simulink model "PubIfDecisionTOS_MDL"  (R2020b)
settings: configuration reference "DspaceConfig" (kept outside this file)
PostLoadFcn:
  | if any(exist('dsrtsu_mdlpostloadfcn', 'file') ~= 0), dsrtsu_mdlpostloadfcn('Execute', bdroot); end
InitFcn:
  | , if any(exist('dsmpb_private', 'file') ~= 0), dsmpb_private('dsmpb_mdlclblib', 'Init', bdroot); end,
undefined symbols (not defined in the file or in its folder): C_TOS_ACCEgoRAxletoFbumplength_m, C_TOS_ACCTargetFront_Flag, C_TOS_AEBJAPedObjDxThre_Val, C_TOS_AEBJAPedObjDyThre_Val, C_TOS_AEBJATargetSize_Val, C_TOS_AEBJAVehObjDxThre_Val, C_TOS_AEBJAVehObjDyThre_Val, C_TOS_AEBJuncPedTargetSize_Val, C_TOS_AEBLatObjDxThre_Val, C_TOS_AEBLatPedDyThre_Val, C_TOS_AEBLatTargetSize_Val, C_TOS_AEBLongTargetInEgoFront_Flag, C_TOS_axAbsGround_Parameter, C_TOS_CameraConfirmedFlag, C_TOS_CNsubjWidth, C_TOS_CurrentLaneCoreMinWidth_Val, C_TOS_CutInProb_Val_Zero, C_TOS_CutOutProb_Val_Zero, C_TOS_D2R_Val, C_TOS_DefaultValueObjectToCenterLine_dy, C_TOS_EgoCarWidth_Val, C_TOS_EgoDxRefPoint_m, C_TOS_EgoRAxletoFbumplength_m, C_TOS_HalfWidthVehicle_Con, C_TOS_HWA_CurrentLaneFlag, C_TOS_HWA_LeftLaneFlag, C_TOS_HWA_MovingDir_Vaild, C_TOS_HWA_MovState_Vaild, C_TOS_HWA_RightLaneFlag, C_TOS_LaneLineCourseErrorFront, C_TOS_LaneLineCourseErrorRear, C_TOS_MotorbikeDefaultWidth_m, C_TOS_NumberOfEffectiveTargets, C_TOS_Obj_Age_Val, C_TOS_Objdx_Constraint_Val, C_TOS_ObjectDefaultWidth_m, C_TOS_ObjInCurrentLane_Val, C_TOS_ObjInCurrentLaneValid, C_TOS_ObjInLeftLaneValid, C_TOS_ObjInRightLaneValid, C_TOS_ObjNotInCurrentLane_Val, C_TOS_ObjNotREElementType, C_TOS_ObjPredictDis_dy_ConstantVal_Zeros, C_TOS_ObjToCenterLine_ConstantVal_Zeros, C_TOS_OFMObjIDInvilad_Val, C_TOS_PIL_LatDisCons_Val_zero, C_TOS_PIL_ObjectCutInFlag_b, C_TOS_PIL_ObjectCutOutFlag_b, C_TOS_PIL_ObjLaneProb_al_Val, C_TOS_PP_ObjFusType_FC_Confirm_b, C_TOS_PP_ObjFusType_FC_FR_Confirm_b, C_TOS_PP_ObjFusType_FR_Confirm_b, C_TOS_RE_80BoolDefault_Val, C_TOS_RE_80Single181Default_Val, C_TOS_RE_80Single255Default_Val, C_TOS_RE_80Uint8Default_Val, C_TOS_RE_D2R, C_TOS_RE_D_180_Val, C_TOS_RE_InvalidObjectID_Val, C_TOS_RE_InvalidTargetChainDir_Val ... (+142)
libraries: simulink x1650, TOS_LIB x361, canfdmsglib x14
(part 29 of 69)

== system PubIfDecisionTOS_MDL/TOS_20201112/TOS_2012080320/TOS/AEB/TOS_AEBJunct_20201208/AEBJunc_Object_Condition1/AEBJA_TargetCondition/TOS_AEBJunc_TargetsCondition ==
  Object_ID : Inport
  PP_ObjFusType_FC_FR_Confirm : Inport  Port=2
  PP_ObjFusType_FR_Confirm : Inport  Port=3
  ObjectType : Inport  Port=4
  Object_Dx : Inport  Port=5
  Object_Dy : Inport  Port=6
  PP_ObjMovingDirSignalProcessing : Inport  Port=7
  Object_HeadingAngle : Inport  Port=8
  Object_VX : Inport  Port=9
  Object_VY : Inport  Port=10
  VIE_EgoVelocity : Inport  Port=11
  psiDtOpt : Inport  Port=12
  axvRefMs2 : Inport  Port=13
  Object_MovingState : Inport  Port=14
  AEBJunc_Target_ObjectID_K1 : Inport  Port=15
  AEBJunc_Target_ObjectType_K1 : Inport  Port=16
  Action Port : ActionPort
  AEBJunc_PedTargetCondition : Subsystem
  AEBJunc_VehTargetCondition : Subsystem
  Bus Creator : BusCreator  Inputs=16
  Bus Selector : BusSelector  OutputSignals=Object_ID,PP_ObjFusType_FC_FR_Confirm,PP_ObjFusType_FR_Confirm,ObjectType,Object_Dx,Object_Dy,PP_ObjMovingDirSignalProcessing,Object_HeadingAngle,Object_VX,Object_VY,VIE_EgoVelocity,psiDtOpt,axvRefMs2,AEBJunc_Target_ObjectID_K1,AEBJunc_Target_ObjectType_K1
  Bus Selector1 : BusSelector  OutputSignals=Object_ID,PP_ObjFusType_FC_FR_Confirm,PP_ObjFusType_FR_Confirm,ObjectType,Object_Dx,Object_Dy,PP_ObjMovingDirSignalProcessing,Object_HeadingAngle,Object_VX,Object_VY,VIE_EgoVelocity,psiDtOpt,axvRefMs2,AEBJunc_Target_ObjectID_K1,AEBJunc_Target_ObjectType_K1,Object_MovingState
  TOS_AEBJunc_PedTargetsDx : Outport
  TOS_AEBJunc_VehTargetsDx : Outport  Port=2
  AEBJunc_PedTargetFusionType_observal : Outport  Port=3
  AEBJunc_PedTargetObjectType_observal : Outport  Port=4
  AEBJunc_PedTargetDXDY_observal : Outport  Port=5
  AEBJunc_PedTargetMovDir_observal : Outport  Port=6
  AEBJunc_VehTargetFusionType_observal : Outport  Port=7
  AEBJunc_VehTargetObjectType_observal : Outport  Port=8
  AEBJunc_VehTargetDXDY_observal : Outport  Port=9
  AEBJunc_VehTargetMovDir_observal : Outport  Port=10
  AEBJunc_VehTargetMovState_observal : Outport  Port=11
  wires:
  AEBJunc_VehTargetCondition/6(AEBJunc_VehTargetMovState_observal) -> AEBJunc_VehTargetMovState_observal/1
  Bus Selector1/16 -> AEBJunc_VehTargetCondition/16(Object_MovingState)  "<Object_MovingState>"
  Object_MovingState/1 -> Bus Creator/14  "Object_MovingState"
  AEBJunc_VehTargetCondition/1(TOS_AEBJunc_VehTargetsDx) -> TOS_AEBJunc_VehTargetsDx/1
  AEBJunc_VehTargetCondition/2(AEBJunc_VehTargetFusionType_observal) -> AEBJunc_VehTargetFusionType_observal/1
  AEBJunc_VehTargetCondition/3(AEBJunc_VehTargetObjectType_observal) -> AEBJunc_VehTargetObjectType_observal/1
  AEBJunc_VehTargetCondition/4(AEBJunc_VehTargetDXDY_observal) -> AEBJunc_VehTargetDXDY_observal/1
  AEBJunc_VehTargetCondition/5(AEBJunc_VehTargetMovDir_observal) -> AEBJunc_VehTargetMovDir_observal/1
  Bus Selector1/1 -> AEBJunc_VehTargetCondition/1(Object_ID)  "<Object_ID>"
  Bus Selector1/2 -> AEBJunc_VehTargetCondition/2(PP_ObjFusType_FC_FR_Confirm)  "<PP_ObjFusType_FC_FR_Confirm>"
  Bus Selector1/3 -> AEBJunc_VehTargetCondition/3(PP_ObjFusType_FR_Confirm)  "<PP_ObjFusType_FR_Confirm>"
  Bus Selector1/4 -> AEBJunc_VehTargetCondition/4(ObjectType)  "<ObjectType>"
  Bus Selector1/5 -> AEBJunc_VehTargetCondition/5(Object_Dx)  "<Object_Dx>"
  Bus Selector1/6 -> AEBJunc_VehTargetCondition/6(Object_Dy)  "<Object_Dy>"
  Bus Selector1/7 -> AEBJunc_VehTargetCondition/7(PP_ObjMovingDirSignalProcessing)  "<PP_ObjMovingDirSignalProcessing>"
  Bus Selector1/8 -> AEBJunc_VehTargetCondition/8(Object_HeadingAngle)  "<Object_HeadingAngle>"
  Bus Selector1/9 -> AEBJunc_VehTargetCondition/9(Object_VX)  "<Object_VX>"
  Bus Selector1/10 -> AEBJunc_VehTargetCondition/10(Object_VY)  "<Object_VY>"
  Bus Selector1/11 -> AEBJunc_VehTargetCondition/11(VIE_EgoVelocity)  "<VIE_EgoVelocity>"
  Bus Selector1/12 -> AEBJunc_VehTargetCondition/12(psiDtOpt)  "<psiDtOpt>"
  Bus Selector1/13 -> AEBJunc_VehTargetCondition/13(axvRefMs2)  "<axvRefMs2>"
  Bus Selector1/14 -> AEBJunc_VehTargetCondition/14(AEBJunc_VehTarget_ObjectID_K1)  "<AEBJunc_Target_ObjectID_K1>"
  Bus Selector1/15 -> AEBJunc_VehTargetCondition/15(AEBJunc_Target_ObjectType_K1)  "<AEBJunc_Target_ObjectType_K1>"
  Bus Selector/15 -> AEBJunc_PedTargetCondition/15(AEBJunc_Target_ObjectType_K1)  "<AEBJunc_Target_ObjectType_K1>"
  Bus Selector/14 -> AEBJunc_PedTargetCondition/14(AEBJunc_PedTarget_ObjectID_K1)  "<AEBJunc_Target_ObjectID_K1>"
  Bus Selector/13 -> AEBJunc_PedTargetCondition/13(axvRefMs2)  "<axvRefMs2>"
  Bus Selector/12 -> AEBJunc_PedTargetCondition/12(psiDtOpt)  "<psiDtOpt>"
  Bus Selector/11 -> AEBJunc_PedTargetCondition/11(VIE_EgoVelocity)  "<VIE_EgoVelocity>"
  Bus Selector/10 -> AEBJunc_PedTargetCondition/10(Object_VY)  "<Object_VY>"
  Bus Selector/9 -> AEBJunc_PedTargetCondition/9(Object_VX)  "<Object_VX>"
  Bus Selector/8 -> AEBJunc_PedTargetCondition/8(Object_HeadingAngle)  "<Object_HeadingAngle>"
  Bus Selector/7 -> AEBJunc_PedTargetCondition/7(PP_ObjMovingDirSignalProcessing)  "<PP_ObjMovingDirSignalProcessing>"
  Bus Selector/6 -> AEBJunc_PedTargetCondition/6(Object_Dy)  "<Object_Dy>"
  Bus Selector/5 -> AEBJunc_PedTargetCondition/5(Object_Dx)  "<Object_Dx>"
  Bus Selector/4 -> AEBJunc_PedTargetCondition/4(ObjectType)  "<ObjectType>"
  Bus Selector/3 -> AEBJunc_PedTargetCondition/3(PP_ObjFusType_FR_Confirm)  "<PP_ObjFusType_FR_Confirm>"
  Bus Selector/2 -> AEBJunc_PedTargetCondition/2(PP_ObjFusType_FC_FR_Confirm)  "<PP_ObjFusType_FC_FR_Confirm>"
  Bus Selector/1 -> AEBJunc_PedTargetCondition/1(Object_ID)  "<Object_ID>"
  Bus Creator/1 -> Bus Selector/1, Bus Selector1/1
  AEBJunc_Target_ObjectType_K1/1 -> Bus Creator/16  "AEBJunc_Target_ObjectType_K1"
  AEBJunc_Target_ObjectID_K1/1 -> Bus Creator/15  "AEBJunc_Target_ObjectID_K1"
  axvRefMs2/1 -> Bus Creator/13  "axvRefMs2"
  psiDtOpt/1 -> Bus Creator/12  "psiDtOpt"
  VIE_EgoVelocity/1 -> Bus Creator/11  "VIE_EgoVelocity"
  Object_VY/1 -> Bus Creator/10  "Object_VY"
  Object_VX/1 -> Bus Creator/9  "Object_VX"
  Object_HeadingAngle/1 -> Bus Creator/8  "Object_HeadingAngle"
  PP_ObjMovingDirSignalProcessing/1 -> Bus Creator/7  "PP_ObjMovingDirSignalProcessing"
  Object_Dy/1 -> Bus Creator/6  "Object_Dy"
  Object_Dx/1 -> Bus Creator/5  "Object_Dx"
  ObjectType/1 -> Bus Creator/4  "ObjectType"
  PP_ObjFusType_FR_Confirm/1 -> Bus Creator/3  "PP_ObjFusType_FR_Confirm"
  PP_ObjFusType_FC_FR_Confirm/1 -> Bus Creator/2  "PP_ObjFusType_FC_FR_Confirm"
  Object_ID/1 -> Bus Creator/1  "Object_ID"
  AEBJunc_PedTargetCondition/5(AEBJunc_PedTargetMovDir_observal) -> AEBJunc_PedTargetMovDir_observal/1
  AEBJunc_PedTargetCondition/4(AEBJunc_PedTargetDXDY_observal) -> AEBJunc_PedTargetDXDY_observal/1
  AEBJunc_PedTargetCondition/3(AEBJunc_PedTargetObjectType_observal) -> AEBJunc_PedTargetObjectType_observal/1
  AEBJunc_PedTargetCondition/2(AEBJunc_PedTargetFusionType_observal) -> AEBJunc_PedTargetFusionType_observal/1
  AEBJunc_PedTargetCondition/1(TOS_AEBJunc_PedTargetsDx) -> TOS_AEBJunc_PedTargetsDx/1

== system PubIfDecisionTOS_MDL/TOS_20201112/TOS_2012080320/TOS/AEB/TOS_AEBJunct_20201208/AEBJunc_Object_Condition1/AEBJA_TargetCondition/TOS_AEBJunc_TargetsConditionDefault ==
  Action Port : ActionPort
  Constant{1,3..5,7..11} (9 alike) : Constant  Value=0  OutDataTypeStr=boolean
  Constant2 : Constant  Value=255  OutDataTypeStr=single
  Constant6 : Constant  Value=255  OutDataTypeStr=single
  TOS_AEBJunc_PedTargetsDx : Outport
  TOS_AEBJunc_VehTargetsDx : Outport  Port=2
  AEBJunc_PedTargetFusionType_observal : Outport  Port=3
  AEBJunc_PedTargetObjectType_observal : Outport  Port=4
  AEBJunc_PedTargetDXDY_observal : Outport  Port=5
  AEBJunc_PedTargetMovDir_observal : Outport  Port=6
  AEBJunc_VehTargetFusionType_observal : Outport  Port=7
  AEBJunc_VehTargetObjectType_observal : Outport  Port=8
  AEBJunc_VehTargetDXDY_observal : Outport  Port=9
  AEBJunc_VehTargetMovDir_observal : Outport  Port=10
  AEBJunc_VehTargetMovState_observal : Outport  Port=11
  wires:
  Constant11/1 -> AEBJunc_VehTargetMovState_observal/1
  Constant8/1 -> AEBJunc_VehTargetObjectType_observal/1
  Constant7/1 -> AEBJunc_VehTargetFusionType_observal/1
  Constant9/1 -> AEBJunc_VehTargetDXDY_observal/1
  Constant10/1 -> AEBJunc_VehTargetMovDir_observal/1
  Constant6/1 -> TOS_AEBJunc_VehTargetsDx/1
  Constant5/1 -> AEBJunc_PedTargetMovDir_observal/1
  Constant4/1 -> AEBJunc_PedTargetDXDY_observal/1
  Constant1/1 -> AEBJunc_PedTargetFusionType_observal/1
  Constant3/1 -> AEBJunc_PedTargetObjectType_observal/1
  Constant2/1 -> TOS_AEBJunc_PedTargetsDx/1

== system PubIfDecisionTOS_MDL/TOS_20201112/TOS_2012080320/TOS/AEB/TOS_AEBJunct_20201208/AEBJunctionTargetInfor/AEBJuncTargetObjectType/AEBJuncTargetObjectType ==
  TOS_AEBJuncTrg_Index : Inport  OutDataTypeStr=uint8
  OFM_SignalVerification : Inport  Port=2
  AEBJunc_Target_ObjectID_K1 : Inport  Port=3
  AEBJunc_Target_ObjectType_K1 : Inport  Port=4
  Action Port : ActionPort  ActionPortLabel=else
  Bus Selector1 : BusSelector  OutputSignals=Object_Type,Object_ID
  Data Type Conversion : DataTypeConversion  OutDataTypeStr=Enum: OFM_OBJ_TYPE_E
  Data Type Conversion1 : DataTypeConversion  OutDataTypeStr=uint8
  Data Type Conversion2 : DataTypeConversion  OutDataTypeStr=Enum: OFM_OBJ_TYPE_E
  Selector : Selector  InputPortWidth=80  IndexOptions=Index vector (port)  Indices=[1 3]  OutputSizes=1
  Selector1 : Selector  InputPortWidth=80  IndexOptions=Index vector (port)  Indices=[1 3]  OutputSizes=1
  TOS_AEBJunc_TargetObjectType : Stateflow chart  TreatAsAtomicUnit=on
  AEBLat_TargetObjectType : Outport
  wires:
  TOS_AEBJuncTrg_Index/1 -> Selector1/2, Selector/2
  Data Type Conversion/1 -> TOS_AEBJunc_TargetObjectType/1(ObjectType)  "Object_Type"
  Selector/1 -> Data Type Conversion/1
  OFM_SignalVerification/1 -> Bus Selector1/1
  Bus Selector1/1 -> Selector/1  "<Object_Type>"
  Data Type Conversion1/1 -> AEBLat_TargetObjectType/1
  AEBJunc_Target_ObjectType_K1/1 -> Data Type Conversion2/1
  Selector1/1 -> TOS_AEBJunc_TargetObjectType/2(Object_ID)  "Object_ID"
  Data Type Conversion2/1 -> TOS_AEBJunc_TargetObjectType/3(AEBJunc_Target_ObjectType_K1)  "AEBJunc_Target_ObjectType_K1"
  AEBJunc_Target_ObjectID_K1/1 -> TOS_AEBJunc_TargetObjectType/4(AEBJunc_Target_ObjectID_K1)  "AEBJunc_Target_ObjectID_K1"
  TOS_AEBJunc_TargetObjectType/1(AEBJunc_TargetObjectType) -> Data Type Conversion1/1  "AEBJunc_TargetObjectType"
  Bus Selector1/2 -> Selector1/1  "<Object_ID>"

== system PubIfDecisionTOS_MDL/TOS_20201112/TOS_2012080320/TOS/AEB/TOS_AEBJunct_20201208/AEBJunctionTargetInfor/AEBJuncTargetObjectType/AEBJuncTargetObjectTypeDefault ==
  Action Port : ActionPort  ActionPortLabel=if(u1)
  Constant : Constant  Value=0  OutDataTypeStr=uint8
  TOS_AEBJuncTargetObjectType : Outport
  wires:
  Constant/1 -> TOS_AEBJuncTargetObjectType/1

== system PubIfDecisionTOS_MDL/TOS_20201112/TOS_2012080320/TOS/AEB/TOS_AEBLatCro1105/AEBLatTrgInfor/AEBLatTargetObjectType/AEBLatTargetObjectType ==
  TOS_AEBLatTrg_Index : Inport  OutDataTypeStr=uint8
  OFM_SignalVerification : Inport  Port=2
  AEBLat_Target_ObjectID_K1 : Inport  Port=3
  AEBLat_Target_ObjectType_K1 : Inport  Port=4
  Action Port : ActionPort
  Bus Selector1 : BusSelector  OutputSignals=Object_ID,Object_Type
  Data Type Conversion : DataTypeConversion  OutDataTypeStr=Enum: OFM_OBJ_TYPE_E
  Data Type Conversion1 : DataTypeConversion  OutDataTypeStr=uint8
  Data Type Conversion2 : DataTypeConversion  OutDataTypeStr=Enum: OFM_OBJ_TYPE_E
  Selector : Selector  InputPortWidth=80  IndexOptions=Index vector (port)  Indices=[1 3]  OutputSizes=1
  Selector1 : Selector  InputPortWidth=80  IndexOptions=Index vector (port)  Indices=[1 3]  OutputSizes=1
  TOS_AEBLat_TargetObjectType : Stateflow chart  TreatAsAtomicUnit=on
  AEBLat_TargetObjectType : Outport
  wires:
  TOS_AEBLatTrg_Index/1 -> Selector1/2, Selector/2
  Data Type Conversion/1 -> TOS_AEBLat_TargetObjectType/2(ObjectType)  "Object_Type"
  Selector/1 -> Data Type Conversion/1
  OFM_SignalVerification/1 -> Bus Selector1/1
  Bus Selector1/2 -> Selector/1  "<Object_Type>"
  Data Type Conversion1/1 -> AEBLat_TargetObjectType/1
  AEBLat_Target_ObjectType_K1/1 -> Data Type Conversion2/1
  Selector1/1 -> TOS_AEBLat_TargetObjectType/1(Object_ID)  "Object_ID"
  Data Type Conversion2/1 -> TOS_AEBLat_TargetObjectType/3(AEBLat_Target_ObjectType_K1)  "AEBLat_Target_ObjectType_K1"
  AEBLat_Target_ObjectID_K1/1 -> TOS_AEBLat_TargetObjectType/4(AEBLat_Target_ObjectID_K1)  "AEBLat_Target_ObjectID_K1"
  TOS_AEBLat_TargetObjectType/1(AEBLat_TargetObjectType) -> Data Type Conversion1/1  "AEBLat_TargetObjectType"
  Bus Selector1/1 -> Selector1/1  "<Object_ID>"

== system PubIfDecisionTOS_MDL/TOS_20201112/TOS_2012080320/TOS/AEB/TOS_AEBLatCro1105/AEBLatTrgInfor/AEBLatTargetObjectType/AEBLatTargetObjectTypeDefault ==
  Action Port : ActionPort
  Constant : Constant  Value=0  OutDataTypeStr=uint8
  TOS_AEBLatTargetObjectType : Outport
  wires:
  Constant/1 -> TOS_AEBLatTargetObjectType/1

== system PubIfDecisionTOS_MDL/TOS_20201112/TOS_2012080320/TOS/AEB/TOS_AEBLatCro1105/AEBLat_Object_Condition/AEBLat_TargetCondition/TOS_AEBLat_TargetsDx ==
  note: 过滤静止目标
  Object_ID : Inport
  PP_ObjFusType_FC_FR_Confirm : Inport  Port=2
  PP_ObjFusType_FR_Confirm : Inport  Port=3
  ObjectType : Inport  Port=4
  Object_Dx : Inport  Port=5
  Object_Dy : Inport  Port=6
  PP_ObjMovingDirSignalProcessing : Inport  Port=7
  Object_HeadingAngle : Inport  Port=8
  Object_VX : Inport  Port=9
  Object_VY : Inport  Port=10
  VIE_EgoVelocity : Inport  Port=11
  psiDtOpt : Inport  Port=12
  AEBLat_Target_ObjectID_K1 : Inport  Port=13
  Action Port : ActionPort
  AEBLat_TargetADxDyArea : Subsystem
  AEBLat_TargetFusionTypeJudge : Subsystem
  AEBLat_TargetObjectTypeFlag : Subsystem
  Chart : Stateflow chart  TreatAsAtomicUnit=on
  Compare To Constant : simulink/Logic and Bit Operations/Compare To Constant  relop===  const=true  OutDataTypeStr=boolean
  Logical Operator : Logic  Inputs=4  AllPortsSameDT=off  OutDataTypeStr=boolean
  TOS_AEBLat_TargetMoveDir : Subsystem
  TOS_AEBLat_TargetsDx : Outport
  AEBLat_TargetFusionType_observal : Outport  Port=2
  AEBLat_TargetObjectType_observal : Outport  Port=3
  AEBLat_TargetDXDY_observal : Outport  Port=4
  AEBLat_TargetMovDir_observal : Outport  Port=5
  wires:
  PP_ObjFusType_FC_FR_Confirm/1 -> AEBLat_TargetFusionTypeJudge/1(PP_ObjFusType_FC_FR_Confirm)
  Object_VY/1 -> [Object_Vy], TOS_AEBLat_TargetMoveDir/5(Object_VY)
  PP_ObjMovingDirSignalProcessing/1 -> TOS_AEBLat_TargetMoveDir/2(PP_ObjMovingDirSignalProcessing)
  Object_HeadingAngle/1 -> TOS_AEBLat_TargetMoveDir/3(Object_HeadingAngle)
  PP_ObjFusType_FR_Confirm/1 -> AEBLat_TargetFusionTypeJudge/2(PP_ObjFusType_FR_Confirm)
  Object_VX/1 -> TOS_AEBLat_TargetMoveDir/4(Object_VX)
  VIE_EgoVelocity/1 -> TOS_AEBLat_TargetMoveDir/6(VIE_EgoVelocity)
  AEBLat_TargetFusionTypeJudge/1(AEBLong_TargetFusionTypeFlag) -> [AEBLong_TargetFusionTypeFlag], Logical Operator/1
  ObjectType/1 -> AEBLat_TargetObjectTypeFlag/1(ObjectType)
  AEBLat_TargetObjectTypeFlag/1(AEBLat_TargetObjectTypeFlag) -> [AEBLat_TargetObjectTypeFlag], Logical Operator/2
  AEBLat_TargetADxDyArea/1(TOS_AEBLat_DxDyAreaFlag) -> Logical Operator/3, [TOS_AEBLat_DxDyAreaFlag]
  TOS_AEBLat_TargetMoveDir/1(TOS_AEBLatTargetMovDirFlg) -> [TOS_AEBLatTargetMovDirFlg], Logical Operator/4  "TOS_AEBLat_TargetMovDir"
  Object_Dy/1 -> TOS_AEBLat_TargetMoveDir/1(Object_Dy), AEBLat_TargetADxDyArea/2(Object_Dy)
  Chart/1(TOS_AEBLat_TargetsDx) -> TOS_AEBLat_TargetsDx/1
  Object_Dx/1 -> AEBLat_TargetADxDyArea/1(Object_Dx), [Object_Dx]
  [AEBLong_TargetFusionTypeFlag] -> AEBLat_TargetFusionType_observal/1
  [AEBLat_TargetObjectTypeFlag] -> AEBLat_TargetObjectType_observal/1
  [TOS_AEBLat_DxDyAreaFlag] -> AEBLat_TargetDXDY_observal/1
  [TOS_AEBLatTargetMovDirFlg] -> AEBLat_TargetMovDir_observal/1
  [AEBLat_Target_ObjectID_K1] -> Chart/4(AEBLat_Target_ObjectID_K1)
  Logical Operator/1 -> Compare To Constant/1
  Compare To Constant/1 -> Chart/1(AEBLat_TargetCondition)
  [Object_Vy] -> Chart/5(Object_Vy)
  psiDtOpt/1 -> Chart/3(psiDtOpt)
  [Object_Dx] -> Chart/6(Object_Dx)
  Object_ID/1 -> AEBLat_TargetObjectTypeFlag/3(ObjectID), [Object_ID]
  [Object_ID] -> Chart/2(Object_ID)
  AEBLat_Target_ObjectID_K1/1 -> [AEBLat_Target_ObjectID_K1], AEBLat_TargetObjectTypeFlag/2(AEBLat_Target_ID_K1)

== system PubIfDecisionTOS_MDL/TOS_20201112/TOS_2012080320/TOS/AEB/TOS_AEBLatCro1105/AEBLat_Object_Condition/AEBLat_TargetCondition/TOS_AEBLat_TargetsDxDefault ==
  Action Port : ActionPort
  Constant{1,3..5} (4 alike) : Constant  Value=0  OutDataTypeStr=boolean
  Constant2 : Constant  Value=255  OutDataTypeStr=single
  TOS_AEBLong_TargetsDx : Outport
  AEBLong_TargetFusionType_observal : Outport  Port=2
  AEBLong_TargetObjectType_observal : Outport  Port=3
  AEBLong_TargetDXDY_observal : Outport  Port=4
  AEBLong_TargetMovDir_observal : Outport  Port=5
  wires:
  Constant2/1 -> TOS_AEBLong_TargetsDx/1
  Constant3/1 -> AEBLong_TargetObjectType_observal/1
  Constant1/1 -> AEBLong_TargetFusionType_observal/1
  Constant4/1 -> AEBLong_TargetDXDY_observal/1
  Constant5/1 -> AEBLong_TargetMovDir_observal/1

== system PubIfDecisionTOS_MDL/TOS_20201112/TOS_2012080320/TOS/AEB/TOS_AEBLatCro1105/AEBLat_Object_Condition2/AEBLat_TargetCondition/TOS_AEBLat_TargetsDx ==
  note: 过滤静止目标
  Object_ID : Inport
  PP_ObjFusType_FC_FR_Confirm : Inport  Port=2
  PP_ObjFusType_FR_Confirm : Inport  Port=3
  ObjectType : Inport  Port=4
  Object_Dx : Inport  Port=5
  Object_Dy : Inport  Port=6
  PP_ObjMovingDirSignalProcessing : Inport  Port=7
  Object_HeadingAngle : Inport  Port=8
  Object_VX : Inport  Port=9
  Object_VY : Inport  Port=10
  VIE_EgoVelocity : Inport  Port=11
  psiDtOpt : Inport  Port=12
  AEBLat_Target_ObjectID_K1 : Inport  Port=13
  Action Port : ActionPort
  AEBLat_TargetADxDyArea : Subsystem
  AEBLat_TargetFusionTypeJudge : Subsystem
  AEBLat_TargetObjectTypeFlag : Subsystem
  Chart : Stateflow chart  TreatAsAtomicUnit=on
  Compare To Constant : simulink/Logic and Bit Operations/Compare To Constant  relop===  const=true  OutDataTypeStr=boolean
  Logical Operator : Logic  Inputs=4  AllPortsSameDT=off  OutDataTypeStr=boolean
  TOS_AEBLat_TargetMoveDir : Subsystem
  TOS_AEBLat_TargetsDx : Outport
  AEBLat_TargetFusionType_observal : Outport  Port=2
  AEBLat_TargetObjectType_observal : Outport  Port=3
  AEBLat_TargetDXDY_observal : Outport  Port=4
  AEBLat_TargetMovDir_observal : Outport  Port=5
  wires:
  PP_ObjFusType_FC_FR_Confirm/1 -> AEBLat_TargetFusionTypeJudge/1(PP_ObjFusType_FC_FR_Confirm)
  Object_VY/1 -> [Object_Vy], TOS_AEBLat_TargetMoveDir/5(Object_VY)
  PP_ObjMovingDirSignalProcessing/1 -> TOS_AEBLat_TargetMoveDir/2(PP_ObjMovingDirSignalProcessing)
  Object_HeadingAngle/1 -> TOS_AEBLat_TargetMoveDir/3(Object_HeadingAngle)
  PP_ObjFusType_FR_Confirm/1 -> AEBLat_TargetFusionTypeJudge/2(PP_ObjFusType_FR_Confirm)
  Object_VX/1 -> TOS_AEBLat_TargetMoveDir/4(Object_VX)
  VIE_EgoVelocity/1 -> TOS_AEBLat_TargetMoveDir/6(VIE_EgoVelocity)
  AEBLat_TargetFusionTypeJudge/1(AEBLong_TargetFusionTypeFlag) -> [AEBLong_TargetFusionTypeFlag], Logical Operator/1
  ObjectType/1 -> AEBLat_TargetObjectTypeFlag/1(ObjectType)
  AEBLat_TargetObjectTypeFlag/1(AEBLat_TargetObjectTypeFlag) -> [AEBLat_TargetObjectTypeFlag], Logical Operator/2
  AEBLat_TargetADxDyArea/1(TOS_AEBLat_DxDyAreaFlag) -> Logical Operator/3, [TOS_AEBLat_DxDyAreaFlag]
  TOS_AEBLat_TargetMoveDir/1(TOS_AEBLatTargetMovDirFlg) -> [TOS_AEBLatTargetMovDirFlg], Logical Operator/4  "TOS_AEBLat_TargetMovDir"
  Object_Dy/1 -> TOS_AEBLat_TargetMoveDir/1(Object_Dy), AEBLat_TargetADxDyArea/2(Object_Dy)
  Chart/1(TOS_AEBLat_TargetsDx) -> TOS_AEBLat_TargetsDx/1
  Object_Dx/1 -> [Object_Dx], AEBLat_TargetADxDyArea/1(Object_Dx)
  [AEBLong_TargetFusionTypeFlag] -> AEBLat_TargetFusionType_observal/1
  [AEBLat_TargetObjectTypeFlag] -> AEBLat_TargetObjectType_observal/1
  [TOS_AEBLat_DxDyAreaFlag] -> AEBLat_TargetDXDY_observal/1
  [TOS_AEBLatTargetMovDirFlg] -> AEBLat_TargetMovDir_observal/1
  Object_ID/1 -> Chart/2(Object_ID)
  AEBLat_Target_ObjectID_K1/1 -> Chart/4(AEBLat_Target_ObjectID_K1)
  Logical Operator/1 -> Compare To Constant/1
  Compare To Constant/1 -> Chart/1(AEBLat_TargetCondition)
  [Object_Vy] -> Chart/5(Object_Vy)
  psiDtOpt/1 -> Chart/3(psiDtOpt)
  [Object_Dx] -> Chart/6(Object_Dx)

== system PubIfDecisionTOS_MDL/TOS_20201112/TOS_2012080320/TOS/AEB/TOS_AEBLatCro1105/AEBLat_Object_Condition2/AEBLat_TargetCondition/TOS_AEBLat_TargetsDxDefault ==
  Action Port : ActionPort
  Constant{1,3..5} (4 alike) : Constant  Value=0  OutDataTypeStr=boolean
  Constant2 : Constant  Value=255  OutDataTypeStr=single
  TOS_AEBLong_TargetsDx : Outport
  AEBLong_TargetFusionType_observal : Outport  Port=2
  AEBLong_TargetObjectType_observal : Outport  Port=3
  AEBLong_TargetDXDY_observal : Outport  Port=4
  AEBLong_TargetMovDir_observal : Outport  Port=5
  wires:
  Constant2/1 -> TOS_AEBLong_TargetsDx/1
  Constant3/1 -> AEBLong_TargetObjectType_observal/1
  Constant1/1 -> AEBLong_TargetFusionType_observal/1
  Constant4/1 -> AEBLong_TargetDXDY_observal/1
  Constant5/1 -> AEBLong_TargetMovDir_observal/1

== system PubIfDecisionTOS_MDL/TOS_20201112/TOS_2012080320/TOS/AEB/TOS_AEBLatCro_20201208/AEBLatTrgInfor/AEBLatTargetObjectType/AEBLatTargetObjectType ==
  TOS_AEBLatTrg_Index : Inport  OutDataTypeStr=uint8
  OFM_SignalVerification : Inport  Port=2
  AEBLat_Target_ObjectID_K1 : Inport  Port=3
  AEBLat_Target_ObjectType_K1 : Inport  Port=4
  Action Port : ActionPort  ActionPortLabel=else
  Bus Selector1 : BusSelector  OutputSignals=Object_ID,Object_Type
  Data Type Conversion : DataTypeConversion  OutDataTypeStr=Enum: OFM_OBJ_TYPE_E
  Data Type Conversion1 : DataTypeConversion  OutDataTypeStr=uint8
  Data Type Conversion2 : DataTypeConversion  OutDataTypeStr=Enum: OFM_OBJ_TYPE_E
  Selector : Selector  InputPortWidth=80  IndexOptions=Index vector (port)  Indices=[1 3]  OutputSizes=1
  Selector1 : Selector  InputPortWidth=80  IndexOptions=Index vector (port)  Indices=[1 3]  OutputSizes=1
  TOS_AEBLat_TargetObjectType : Stateflow chart  TreatAsAtomicUnit=on
  AEBLat_TargetObjectType : Outport
  wires:
  TOS_AEBLatTrg_Index/1 -> Selector1/2, Selector/2
  Data Type Conversion/1 -> TOS_AEBLat_TargetObjectType/2(ObjectType)  "Object_Type"
  Selector/1 -> Data Type Conversion/1
  OFM_SignalVerification/1 -> Bus Selector1/1
  Bus Selector1/2 -> Selector/1  "<Object_Type>"
  Data Type Conversion1/1 -> AEBLat_TargetObjectType/1
  AEBLat_Target_ObjectType_K1/1 -> Data Type Conversion2/1
  Selector1/1 -> TOS_AEBLat_TargetObjectType/1(Object_ID)  "Object_ID"
  Data Type Conversion2/1 -> TOS_AEBLat_TargetObjectType/3(AEBLat_Target_ObjectType_K1)  "AEBLat_Target_ObjectType_K1"
  AEBLat_Target_ObjectID_K1/1 -> TOS_AEBLat_TargetObjectType/4(AEBLat_Target_ObjectID_K1)  "AEBLat_Target_ObjectID_K1"
  TOS_AEBLat_TargetObjectType/1(AEBLat_TargetObjectType) -> Data Type Conversion1/1  "AEBLat_TargetObjectType"
  Bus Selector1/1 -> Selector1/1  "<Object_ID>"

== system PubIfDecisionTOS_MDL/TOS_20201112/TOS_2012080320/TOS/AEB/TOS_AEBLatCro_20201208/AEBLatTrgInfor/AEBLatTargetObjectType/AEBLatTargetObjectTypeDefault ==
  Action Port : ActionPort  ActionPortLabel=if(u1)
  Constant : Constant  Value=0  OutDataTypeStr=uint8
  TOS_AEBLatTargetObjectType : Outport
  wires:
  Constant/1 -> TOS_AEBLatTargetObjectType/1

== system PubIfDecisionTOS_MDL/TOS_20201112/TOS_2012080320/TOS/AEB/TOS_AEBLatCro_20201208/AEBLat_Object_Condition/AEBLat_TargetCondition/TOS_AEBLat_TargetsDx ==
  note: 过滤静止目标
  Object_ID : Inport
  PP_ObjFusType_FC_FR_Confirm : Inport  Port=2
  PP_ObjFusType_FR_Confirm : Inport  Port=3
  ObjectType : Inport  Port=4
  Object_Dx : Inport  Port=5
  Object_Dy : Inport  Port=6
  PP_ObjMovingDirSignalProcessing : Inport  Port=7
  Object_HeadingAngle : Inport  Port=8
  Object_VX : Inport  Port=9
  Object_VY : Inport  Port=10
  VIE_EgoVelocity : Inport  Port=11
  psiDtOpt : Inport  Port=12
  AEBLat_Target_ObjectID_K1 : Inport  Port=13
  Action Port : ActionPort  ActionPortLabel=else
  AEBLat_TargetADxDyArea : Subsystem
  AEBLat_TargetFusionTypeJudge : Subsystem
  AEBLat_TargetObjectTypeFlag : Subsystem
  Chart : Stateflow chart  TreatAsAtomicUnit=on
  Compare To Constant : simulink/Logic and Bit Operations/Compare To Constant  relop===  const=true  OutDataTypeStr=boolean
  Logical Operator : Logic  Inputs=4  AllPortsSameDT=off  OutDataTypeStr=boolean
  TOS_AEBLat_TargetMoveDir : Subsystem
  TOS_AEBLat_TargetsDx : Outport
  AEBLat_TargetFusionType_observal : Outport  Port=2
  AEBLat_TargetObjectType_observal : Outport  Port=3
  AEBLat_TargetDXDY_observal : Outport  Port=4
  AEBLat_TargetMovDir_observal : Outport  Port=5
  wires:
  PP_ObjFusType_FC_FR_Confirm/1 -> AEBLat_TargetFusionTypeJudge/1(PP_ObjFusType_FC_FR_Confirm)
  Object_VY/1 -> [Object_Vy], TOS_AEBLat_TargetMoveDir/5(Object_VY)
  PP_ObjMovingDirSignalProcessing/1 -> TOS_AEBLat_TargetMoveDir/2(PP_ObjMovingDirSignalProcessing)
  Object_HeadingAngle/1 -> TOS_AEBLat_TargetMoveDir/3(Object_HeadingAngle)
  PP_ObjFusType_FR_Confirm/1 -> AEBLat_TargetFusionTypeJudge/2(PP_ObjFusType_FR_Confirm)
  Object_VX/1 -> TOS_AEBLat_TargetMoveDir/4(Object_VX)
  VIE_EgoVelocity/1 -> TOS_AEBLat_TargetMoveDir/6(VIE_EgoVelocity)
  AEBLat_TargetFusionTypeJudge/1(AEBLong_TargetFusionTypeFlag) -> [AEBLong_TargetFusionTypeFlag], Logical Operator/1
  ObjectType/1 -> AEBLat_TargetObjectTypeFlag/1(ObjectType)
  AEBLat_TargetObjectTypeFlag/1(AEBLat_TargetObjectTypeFlag) -> [AEBLat_TargetObjectTypeFlag], Logical Operator/2
  AEBLat_TargetADxDyArea/1(TOS_AEBLat_DxDyAreaFlag) -> Logical Operator/3, [TOS_AEBLat_DxDyAreaFlag]
  TOS_AEBLat_TargetMoveDir/1(TOS_AEBLatTargetMovDirFlg) -> [TOS_AEBLatTargetMovDirFlg], Logical Operator/4  "TOS_AEBLat_TargetMovDir"
  Object_Dy/1 -> TOS_AEBLat_TargetMoveDir/1(Object_Dy), AEBLat_TargetADxDyArea/2(Object_Dy)
  Chart/1(TOS_AEBLat_TargetsDx) -> TOS_AEBLat_TargetsDx/1
  Object_Dx/1 -> AEBLat_TargetADxDyArea/1(Object_Dx), [Object_Dx]
  [AEBLong_TargetFusionTypeFlag] -> AEBLat_TargetFusionType_observal/1
  [AEBLat_TargetObjectTypeFlag] -> AEBLat_TargetObjectType_observal/1
  [TOS_AEBLat_DxDyAreaFlag] -> AEBLat_TargetDXDY_observal/1
  [TOS_AEBLatTargetMovDirFlg] -> AEBLat_TargetMovDir_observal/1
  [AEBLat_Target_ObjectID_K1] -> Chart/4(AEBLat_Target_ObjectID_K1)
  Logical Operator/1 -> Compare To Constant/1
  Compare To Constant/1 -> Chart/1(AEBLat_TargetCondition)
  [Object_Vy] -> Chart/5(Object_Vy)
  psiDtOpt/1 -> Chart/3(psiDtOpt)
  [Object_Dx] -> Chart/6(Object_Dx)
  Object_ID/1 -> AEBLat_TargetObjectTypeFlag/3(ObjectID), [Object_ID]
  [Object_ID] -> Chart/2(Object_ID)
  AEBLat_Target_ObjectID_K1/1 -> [AEBLat_Target_ObjectID_K1], AEBLat_TargetObjectTypeFlag/2(AEBLat_Target_ID_K1)
  [AEBLat_Target_ObjectID_K1] -> TOS_AEBLat_TargetMoveDir/7(AEBLat_Target_ID_K1)
  [Object_ID] -> TOS_AEBLat_TargetMoveDir/8(ObjectID)

== system PubIfDecisionTOS_MDL/TOS_20201112/TOS_2012080320/TOS/AEB/TOS_AEBLatCro_20201208/AEBLat_Object_Condition/AEBLat_TargetCondition/TOS_AEBLat_TargetsDxDefault ==
  Action Port : ActionPort  ActionPortLabel=if(u1 ~= 0)
  Constant{1,3..5} (4 alike) : Constant  Value=0  OutDataTypeStr=boolean
  Constant2 : Constant  Value=255  OutDataTypeStr=single
  TOS_AEBLong_TargetsDx : Outport
  AEBLong_TargetFusionType_observal : Outport  Port=2
  AEBLong_TargetObjectType_observal : Outport  Port=3
  AEBLong_TargetDXDY_observal : Outport  Port=4
  AEBLong_TargetMovDir_observal : Outport  Port=5
  wires:
  Constant2/1 -> TOS_AEBLong_TargetsDx/1
  Constant3/1 -> AEBLong_TargetObjectType_observal/1
  Constant1/1 -> AEBLong_TargetFusionType_observal/1
  Constant4/1 -> AEBLong_TargetDXDY_observal/1
  Constant5/1 -> AEBLong_TargetMovDir_observal/1

== system PubIfDecisionTOS_MDL/TOS_20201112/TOS_2012080320/TOS/AEB/TOS_AEBLatCro_20201208/AEBLat_Object_Condition2/AEBLat_TargetCondition/TOS_AEBLat_TargetsDx ==
  note: 过滤静止目标
  Object_ID : Inport
  PP_ObjFusType_FC_FR_Confirm : Inport  Port=2
  PP_ObjFusType_FR_Confirm : Inport  Port=3
  ObjectType : Inport  Port=4
  Object_Dx : Inport  Port=5
  Object_Dy : Inport  Port=6
  PP_ObjMovingDirSignalProcessing : Inport  Port=7
  Object_HeadingAngle : Inport  Port=8
  Object_VX : Inport  Port=9
  Object_VY : Inport  Port=10
  VIE_EgoVelocity : Inport  Port=11
  psiDtOpt : Inport  Port=12
  AEBLat_Target_ObjectID_K1 : Inport  Port=13
  Action Port : ActionPort
  AEBLat_TargetADxDyArea : Subsystem
  AEBLat_TargetFusionTypeJudge : Subsystem
  AEBLat_TargetObjectTypeFlag : Subsystem
  Chart : Stateflow chart  TreatAsAtomicUnit=on
  Compare To Constant : simulink/Logic and Bit Operations/Compare To Constant  relop===  const=true  OutDataTypeStr=boolean
  Logical Operator : Logic  Inputs=4  AllPortsSameDT=off  OutDataTypeStr=boolean
  TOS_AEBLat_TargetMoveDir : Subsystem
  TOS_AEBLat_TargetsDx : Outport
  AEBLat_TargetFusionType_observal : Outport  Port=2
  AEBLat_TargetObjectType_observal : Outport  Port=3
  AEBLat_TargetDXDY_observal : Outport  Port=4
  AEBLat_TargetMovDir_observal : Outport  Port=5
  wires:
  PP_ObjFusType_FC_FR_Confirm/1 -> AEBLat_TargetFusionTypeJudge/1(PP_ObjFusType_FC_FR_Confirm)
  Object_VY/1 -> [Object_Vy], TOS_AEBLat_TargetMoveDir/5(Object_VY)
  PP_ObjMovingDirSignalProcessing/1 -> TOS_AEBLat_TargetMoveDir/2(PP_ObjMovingDirSignalProcessing)
  Object_HeadingAngle/1 -> TOS_AEBLat_TargetMoveDir/3(Object_HeadingAngle)
  PP_ObjFusType_FR_Confirm/1 -> AEBLat_TargetFusionTypeJudge/2(PP_ObjFusType_FR_Confirm)
  Object_VX/1 -> TOS_AEBLat_TargetMoveDir/4(Object_VX)
  VIE_EgoVelocity/1 -> TOS_AEBLat_TargetMoveDir/6(VIE_EgoVelocity)
  AEBLat_TargetFusionTypeJudge/1(AEBLong_TargetFusionTypeFlag) -> [AEBLong_TargetFusionTypeFlag], Logical Operator/1
  ObjectType/1 -> AEBLat_TargetObjectTypeFlag/1(ObjectType)
  AEBLat_TargetObjectTypeFlag/1(AEBLat_TargetObjectTypeFlag) -> [AEBLat_TargetObjectTypeFlag], Logical Operator/2
  AEBLat_TargetADxDyArea/1(TOS_AEBLat_DxDyAreaFlag) -> Logical Operator/3, [TOS_AEBLat_DxDyAreaFlag]
  TOS_AEBLat_TargetMoveDir/1(TOS_AEBLatTargetMovDirFlg) -> [TOS_AEBLatTargetMovDirFlg], Logical Operator/4  "TOS_AEBLat_TargetMovDir"
  Object_Dy/1 -> TOS_AEBLat_TargetMoveDir/1(Object_Dy), AEBLat_TargetADxDyArea/2(Object_Dy)
  Chart/1(TOS_AEBLat_TargetsDx) -> TOS_AEBLat_TargetsDx/1
  Object_Dx/1 -> [Object_Dx], AEBLat_TargetADxDyArea/1(Object_Dx)
  [AEBLong_TargetFusionTypeFlag] -> AEBLat_TargetFusionType_observal/1
  [AEBLat_TargetObjectTypeFlag] -> AEBLat_TargetObjectType_observal/1
  [TOS_AEBLat_DxDyAreaFlag] -> AEBLat_TargetDXDY_observal/1
  [TOS_AEBLatTargetMovDirFlg] -> AEBLat_TargetMovDir_observal/1
  Object_ID/1 -> Chart/2(Object_ID)
  AEBLat_Target_ObjectID_K1/1 -> Chart/4(AEBLat_Target_ObjectID_K1)
  Logical Operator/1 -> Compare To Constant/1
  Compare To Constant/1 -> Chart/1(AEBLat_TargetCondition)
  [Object_Vy] -> Chart/5(Object_Vy)
  psiDtOpt/1 -> Chart/3(psiDtOpt)
  [Object_Dx] -> Chart/6(Object_Dx)

== system PubIfDecisionTOS_MDL/TOS_20201112/TOS_2012080320/TOS/AEB/TOS_AEBLatCro_20201208/AEBLat_Object_Condition2/AEBLat_TargetCondition/TOS_AEBLat_TargetsDxDefault ==
  Action Port : ActionPort
  Constant{1,3..5} (4 alike) : Constant  Value=0  OutDataTypeStr=boolean
  Constant2 : Constant  Value=255  OutDataTypeStr=single
  TOS_AEBLong_TargetsDx : Outport
  AEBLong_TargetFusionType_observal : Outport  Port=2
  AEBLong_TargetObjectType_observal : Outport  Port=3
  AEBLong_TargetDXDY_observal : Outport  Port=4
  AEBLong_TargetMovDir_observal : Outport  Port=5
  wires:
  Constant2/1 -> TOS_AEBLong_TargetsDx/1
  Constant3/1 -> AEBLong_TargetObjectType_observal/1
  Constant1/1 -> AEBLong_TargetFusionType_observal/1
  Constant4/1 -> AEBLong_TargetDXDY_observal/1
  Constant5/1 -> AEBLong_TargetMovDir_observal/1

== system PubIfDecisionTOS_MDL/TOS_20201112/TOS_2012080320/TOS/AEB/TOS_AEBLong/AEBLongTargetInfor/AEBLongTargetMovingDir/AEBLongTargetInfroDefault ==
  Action Port : ActionPort  ActionPortLabel=if(u1)
  Constant : Constant  Value=0  OutDataTypeStr=uint8
  TOS_AEBLongTargetMovingDir : Outport
  wires:
  Constant/1 -> TOS_AEBLongTargetMovingDir/1

== system PubIfDecisionTOS_MDL/TOS_20201112/TOS_2012080320/TOS/AEB/TOS_AEBLong/AEBLongTargetInfor/AEBLongTargetMovingDir/AEBLongTargetMovingDir ==
  TOS_AddAttributes : Inport
  TOS_AEBLongTargetIndex : Inport  Port=2
  Action Port : ActionPort  ActionPortLabel=else
  Bus Creator : BusCreator  Inputs=2
  Bus Selector : BusSelector  OutputSignals=TOS_AddAttributes.PP_MovingState_AEB_SignalProcessing,TOS_AEBLongTargetIndex,TOS_AddAttributes.PP_ObjMovingDirSignalProcessing
  Subsystem : Subsystem
  TOS_AEBLongTargetMovingDir : Outport
  wires:
  TOS_AddAttributes/1 -> Bus Creator/1  "TOS_AddAttributes"
  TOS_AEBLongTargetIndex/1 -> Bus Creator/2  "TOS_AEBLongTargetIndex"
  Bus Creator/1 -> Bus Selector/1
  Subsystem/1(TOS_AEBLongTargetMovingDir) -> TOS_AEBLongTargetMovingDir/1
  Bus Selector/2 -> Subsystem/2(AEBLongTargetIndex)  "<TOS_AEBLongTargetIndex>"
  Bus Selector/1 -> Subsystem/1(PP_MovingState)  "<PP_MovingState_AEB_SignalProcessing>"
  Bus Selector/3 -> Subsystem/3(PP_MovingDir)  "<PP_ObjMovingDirSignalProcessing>"

== system PubIfDecisionTOS_MDL/TOS_20201112/TOS_2012080320/TOS/AEB/TOS_AEBLong/AEBLong_Confirm/AEBLong/AEBLong_TrgConfirm ==
  In1 : Inport
  Object_ID : Inport  Port=2
  Object_DX : Inport  Port=3
  Object_ObstacleProb : Inport  Port=4
  Object_ExistProb : Inport  Port=5
  Object_Fus_Type : Inport  Port=6
  object_MovingState : Inport  Port=7
  Object_HeadingAngle : Inport  Port=8
  Object_Type : Inport  Port=9
  VIE_EgoVelocity : Inport  Port=10
  PIL_LeftLaneProb : Inport  Port=11
  PIL_CurrentLaneProb : Inport  Port=12
  PIL_RightLaneProb : Inport  Port=13
  PP_MovingStateSignalProcessing : Inport  Port=14
  PP_ObjMovingDirSignalProcessing : Inport  Port=15
  PP_ObjectToCenterLine_dy : Inport  Port=16
  TLJ_TargetInCLValidityflg : Inport  Port=17
  PP_CurrentLaneWidth : Inport  Port=18
  Object_DY : Inport  Port=19
  SteerWheelAng : Inport  Port=20
  SteerWheelSpd : Inport  Port=21
  PP_ObjFusType_FC_FR_Confirm : Inport  Port=22
  PP_ObjFusType_FR_Confirm : Inport  Port=23
  PP_ObjFusType_FC_Confirm : Inport  Port=24
  Object_VX : Inport  Port=25
  Object_VY : Inport  Port=26
  PIL_OverlapRatio : Inport  Port=27
  AEBLong_Target_ID_K1 : Inport  Port=28
  AEBLong_Target_ID_K2 : Inport  Port=29
  AEBLong_Target_MovState_K1 : Inport  Port=30
  AEBLong_Target_MovState_K2 : Inport  Port=31
  Action Port : ActionPort  ActionPortLabel=else
  AEBLongTrgJudg : Subsystem
  Subsystem : Subsystem
  TOS_AEBLong_TargetConditionJudge : Outport
  TOS_AEBLong_TargetDis_ObserVale : Outport  Port=2
  TOS_AEBLong_ObstacleProb_ObserVale : Outport  Port=3
  TOS_AEBLong_TargetExistProb_ObserVale : Outport  Port=4
  TOS_AEBLong_ObjFusType_ObserVale : Outport  Port=5
  TOS_AEBLong_TargetInEgoFront_ObserVale : Outport  Port=6
  TOS_AEBLong_TargetMovingDir_ObserVale : Outport  Port=7
  TOS_AEB_Stockade_ObserVale : Outport  Port=8
  TOS_AEBLong_TargetDy_ObserVale : Outport  Port=9
  TOS_AEBLong_SteerWheelAngConfirm_ObserVale : Outport  Port=10
  TOS_AEBLong_OverlapRatio_ObserVale : Outport  Port=11
  wires:
  Object_ExistProb/1 -> Subsystem/5(Object_ExistProb)
  Object_ObstacleProb/1 -> Subsystem/4(Object_ObstacleProb)
  Object_DX/1 -> Subsystem/3(Object_DX)
  AEBLongTrgJudg/10(TOS_AEBLong_SteerWheelAngConfirm_ObserVale) -> TOS_AEBLong_SteerWheelAngConfirm_ObserVale/1
  PP_ObjMovingDirSignalProcessing/1 -> Subsystem/15(PP_ObjMovingDirSignalProcessing)
  PP_MovingStateSignalProcessing/1 -> Subsystem/14(PP_MovingStateSignalProcessing)
  PIL_LeftLaneProb/1 -> Subsystem/11(PIL_LeftLaneProb)
  VIE_EgoVelocity/1 -> Subsystem/10(VIE_EgoVelocity)
  Subsystem/11(PILCurrentLaneProb) -> AEBLongTrgJudg/11(PIL_CurrentLaneProb)
  TLJ_TargetInCLValidityflg/1 -> Subsystem/17(TLJ_TargetInCLValidityflg)
  Subsystem/4(ObjectExistProb) -> AEBLongTrgJudg/4(Object_ExistProb)
  AEBLongTrgJudg/8(TOS_AEB_Stockade_ObserVale) -> TOS_AEB_Stockade_ObserVale/1
  Subsystem/2(ObjectDX) -> AEBLongTrgJudg/2(Object_DX)
  Subsystem/8(ObjectType) -> AEBLongTrgJudg/8(Object_Type)
  AEBLongTrgJudg/3(TOS_AEBLong_ObstacleProb_ObserVale) -> TOS_AEBLong_ObstacleProb_ObserVale/1
  Subsystem/14(PPObjMovingDirSignalProcessing) -> AEBLongTrgJudg/14(PP_ObjMovingDirSignalProcessing)
  object_MovingState/1 -> Subsystem/7(object_MovingState)
  AEBLongTrgJudg/4(TOS_AEBLong_TargetExistProb_ObserVale) -> TOS_AEBLong_TargetExistProb_ObserVale/1
  In1/1 -> Subsystem/1(Dx1stNearestObjIndex)
  Subsystem/1(ObjectID) -> AEBLongTrgJudg/1(ObjectID)
  PIL_CurrentLaneProb/1 -> Subsystem/12(PIL_CurrentLaneProb)
  AEBLongTrgJudg/5(TOS_AEBLong_ObjFusType_ObserVale) -> TOS_AEBLong_ObjFusType_ObserVale/1
  PP_CurrentLaneWidth/1 -> Subsystem/18(PP_CurrentLaneWidth)
  AEBLongTrgJudg/7(TOS_AEBLong_TargetMovingDir_ObserVale) -> TOS_AEBLong_TargetMovingDir_ObserVale/1
  Subsystem/12(PILRightLaneProb) -> AEBLongTrgJudg/12(PIL_RightLaneProb)
  Object_ID/1 -> Subsystem/2(Object_ID)
  Subsystem/6(objectMovingState) -> AEBLongTrgJudg/6(object_MovingState)
  SteerWheelAng/1 -> AEBLongTrgJudg/29(SteerWheelAng)
  AEBLongTrgJudg/9(TOS_AEBLong_TargetDy_ObserVale) -> TOS_AEBLong_TargetDy_ObserVale/1
  Subsystem/17(TLJTargetInCLValidityflg) -> AEBLongTrgJudg/17(TLJ_TargetInCLValidityflg)
  Object_DY/1 -> Subsystem/19(Object_DY)
  Object_HeadingAngle/1 -> Subsystem/8(Object_HeadingAngle)
  AEBLongTrgJudg/6(TOS_AEBLong_TargetInEgoFront_ObserVale) -> TOS_AEBLong_TargetInEgoFront_ObserVale/1
  PP_ObjectToCenterLine_dy/1 -> Subsystem/16(PP_ObjectToCenterLine_dy)
  PIL_RightLaneProb/1 -> Subsystem/13(PIL_RightLaneProb)
  AEBLongTrgJudg/2(TOS_AEBLong_TargetDis_ObserVale) -> TOS_AEBLong_TargetDis_ObserVale/1
  Subsystem/5(ObjectFus_Type) -> AEBLongTrgJudg/5(Object_Fus_Type)
  Object_Fus_Type/1 -> Subsystem/6(Object_Fus_Type)
  Subsystem/15(PPObjectToCenterLine_dy) -> AEBLongTrgJudg/15(PP_ObjectToCenterLine_dy)
  Subsystem/7(ObjectHeadingAngle) -> AEBLongTrgJudg/7(Object_HeadingAngle)
  Subsystem/10(PILLeftLaneProb) -> AEBLongTrgJudg/10(PIL_LeftLaneProb)
  Subsystem/3(ObjectObstacleProb) -> AEBLongTrgJudg/3(Object_ObstacleProb)
  AEBLongTrgJudg/1(TOS_AEBLong_TargetConditionJudge) -> TOS_AEBLong_TargetConditionJudge/1
  SteerWheelSpd/1 -> AEBLongTrgJudg/30(SteerWheelSpd)
  Subsystem/9(VIEEgoVelocity) -> AEBLongTrgJudg/9(VIE_EgoVelocity)
  Subsystem/18(ObjectDY) -> AEBLongTrgJudg/18(Object_DY)
  Subsystem/16(PPCurrentLaneWidth) -> AEBLongTrgJudg/16(PP_CurrentLaneWidth)
  Subsystem/13(PPMovingStateSignalProcessing) -> AEBLongTrgJudg/13(PP_MovingStateSignalProcessing)
  Object_Type/1 -> Subsystem/9(Object_Type)
  PP_ObjFusType_FR_Confirm/1 -> Subsystem/21(PP_ObjFusType_FR_Confirm)
  PP_ObjFusType_FC_FR_Confirm/1 -> Subsystem/20(PP_ObjFusType_FC_FR_Confirm)
  PP_ObjFusType_FC_Confirm/1 -> Subsystem/22(PP_ObjFusType_FC_Confirm)
  Subsystem/19(PP_ObjFusType_FC_FR_Confirm_) -> AEBLongTrgJudg/19(PP_ObjFusType_FC_FR_Confirm)
  Subsystem/20(PP_ObjFusType_FR_Confirm_) -> AEBLongTrgJudg/20(PP_ObjFusType_FR_Confirm)
  Subsystem/21(PP_ObjFusType_FC_Confirm_) -> AEBLongTrgJudg/21(PP_ObjFusType_FC_Confirm)
  Object_VX/1 -> Subsystem/23(Object_VX)
  Object_VY/1 -> Subsystem/24(Object_VY)
  Subsystem/22(ObjectVX) -> AEBLongTrgJudg/22(Object_VX)
  Subsystem/23(ObjectVY) -> AEBLongTrgJudg/23(Object_VY)
  Subsystem/24(PILOverlapRatio) -> AEBLongTrgJudg/24(PIL_OverlapRatio)
  PIL_OverlapRatio/1 -> Subsystem/25(PIL_OverlapRatio)
  AEBLongTrgJudg/11(TOS_AEBLong_OverlapRatio_ObserVale) -> TOS_AEBLong_OverlapRatio_ObserVale/1
  AEBLong_Target_ID_K1/1 -> Subsystem/26(AEBLong_Target_ID_K1)  "AEBLong_Target_ID_K1"
  AEBLong_Target_ID_K2/1 -> Subsystem/27(AEBLong_Target_ID_K2)  "AEBLong_Target_ID_K2"
  AEBLong_Target_MovState_K1/1 -> Subsystem/28(AEBLong_Target_MovState_K1)
  AEBLong_Target_MovState_K2/1 -> Subsystem/29(AEBLong_Target_MovState_K2)
  Subsystem/25(AEBLongTarget_ID_K2) -> AEBLongTrgJudg/25(AEBLong_Target_ID_K1)
  Subsystem/26(AEBLongTarget_ID_K1) -> AEBLongTrgJudg/26(AEBLong_Target_ID_K2)
  Subsystem/27(AEBLongTarget_MovState_K2) -> AEBLongTrgJudg/27(AEBLong_Target_MovState_K1)
  Subsystem/28(AEBLongTarget_MovState_K1) -> AEBLongTrgJudg/28(AEBLong_Target_MovState_K2)

== system PubIfDecisionTOS_MDL/TOS_20201112/TOS_2012080320/TOS/AEB/TOS_AEBLong/AEBLong_Confirm/AEBLong/AEBLong_TrgConfirmDefault ==
  Action Port : ActionPort  ActionPortLabel=if(u1 ~= 0)
  Constant{1..11} (11 alike) : Constant  Value=0  OutDataTypeStr=boolean
  TOS_AEBLong_TargetConditionJudge : Outport
  TOS_AEBLong_TargetDis_ObserVale : Outport  Port=2
  TOS_AEBLong_ObstacleProb_ObserVale : Outport  Port=3
  TOS_AEBLong_TargetExistProb_ObserVale : Outport  Port=4
  TOS_AEBLong_ObjFusType_ObserVale : Outport  Port=5
  TOS_AEBLong_TargetInEgoFront_ObserVale : Outport  Port=6
  TOS_AEBLong_TargetMovingDir_ObserVale : Outport  Port=7
  TOS_AEB_Stockade_ObserVale : Outport  Port=8
  TOS_AEBLong_TargetDy_ObserVale : Outport  Port=9
  TOS_AEBLong_SteerWheelAngConfirm_ObserVale : Outport  Port=10
  TOS_AEBLong_OverlapRatio_ObserVale : Outport  Port=11
  wires:
  Constant2/1 -> TOS_AEBLong_TargetConditionJudge/1
  Constant5/1 -> TOS_AEBLong_ObjFusType_ObserVale/1
  Constant1/1 -> TOS_AEBLong_TargetDis_ObserVale/1
  Constant7/1 -> TOS_AEBLong_TargetMovingDir_ObserVale/1
  Constant6/1 -> TOS_AEBLong_TargetInEgoFront_ObserVale/1
  Constant10/1 -> TOS_AEBLong_SteerWheelAngConfirm_ObserVale/1
  Constant3/1 -> TOS_AEBLong_ObstacleProb_ObserVale/1
  Constant4/1 -> TOS_AEBLong_TargetExistProb_ObserVale/1
  Constant8/1 -> TOS_AEB_Stockade_ObserVale/1
  Constant9/1 -> TOS_AEBLong_TargetDy_ObserVale/1
  Constant11/1 -> TOS_AEBLong_OverlapRatio_ObserVale/1

== system PubIfDecisionTOS_MDL/TOS_20201112/TOS_2012080320/TOS/AEB/TOS_AEBLong/AEBLong_Target_PreJudge/AEBLONG_Target_PreFilt/AEBLONG_TargetPreCondJudge ==
  note: 判断是否为护栏目标
  note: 针对，选中目标后，过滤突然出现的纵向距离更近的单雷达静止目标
  Object_ID : Inport
  PP_ObjFusType_FC_FR_Confirm : Inport  Port=2
  PP_ObjFusType_FR_Confirm : Inport  Port=3
  PP_ObjFusType_FC_Confirm : Inport  Port=4
  Obj_MovingState : Inport  Port=5
  Obj_Dx : Inport  Port=6
  Object_ObstacleProb : Inport  Port=7
  Object_DY : Inport  Port=8
  AEBLONG_Target_ID_K1 : Inport  Port=9
  AEBLONG_Target_Dx_K1 : Inport  Port=10
  PP_REElementType : Inport  Port=11
  Action Port : ActionPort  ActionPortLabel=else
  AEBLONGTarget_Fence : Subsystem
  AEBLONGTarget_FusionType : Subsystem
  AEBLONGTarget_PassedbyTarget : Subsystem
  Bus Creator : BusCreator  Inputs=11
  Bus Selector1 : BusSelector  OutputSignals=PP_ObjFusType_FR_Confirm,Obj_MovingState,Obj_Dx,AEBLONG_Target_ID_K1,AEBLONG_Target_Dx_K1,Object_ID
  Bus Selector2 : BusSelector  OutputSignals=PP_ObjFusType_FC_FR_Confirm,PP_ObjFusType_FC_Confirm
  Bus Selector3 : BusSelector  OutputSignals=PP_ObjFusType_FR_Confirm,Obj_MovingState,Object_ObstacleProb,Object_DY
  Bus Selector7 : BusSelector  OutputSignals=PP_REElementType
  Logical Operator : Logic  Operator=NOT  AllPortsSameDT=off  OutDataTypeStr=boolean
  Logical Operator2 : Logic  Operator=NOT  AllPortsSameDT=off  OutDataTypeStr=boolean
  Logical Operator3 : Logic  Inputs=4  AllPortsSameDT=off  OutDataTypeStr=boolean
  REElementType : Subsystem
  TOS_AEBLONG_Target_PreFiltFlag : Outport
  TOS_AEBLONG_Target_FusionTypeFlag_ObserVale : Outport  Port=2
  TOS_AEBLONG_Target_PassedbyTarget_Flag_ObserVale : Outport  Port=3
  TOS_AEBLONG_Target_FenceFlag_ObserVale : Outport  Port=4
  TOS_AEBLONG_Target_REElementType_ObserVale : Outport  Port=5
  wires:
  AEBLONGTarget_FusionType/1(TOS_AEBLONG_Target_FusionTypeFlag) -> Logical Operator3/1, TOS_AEBLONG_Target_FusionTypeFlag_ObserVale/1
  AEBLONGTarget_PassedbyTarget/1(TOS_AEBLONG_Target_PassedbyTarget_Flag) -> Logical Operator/1
  AEBLONGTarget_Fence/1(TOS_AEBLONG_Target_FenceFlag) -> Logical Operator2/1
  Logical Operator2/1 -> Logical Operator3/3, TOS_AEBLONG_Target_FenceFlag_ObserVale/1
  Logical Operator/1 -> Logical Operator3/2, TOS_AEBLONG_Target_PassedbyTarget_Flag_ObserVale/1
  Logical Operator3/1 -> TOS_AEBLONG_Target_PreFiltFlag/1
  Bus Selector1/6 -> AEBLONGTarget_PassedbyTarget/6(Object_ID)  "<Object_ID>"
  PP_ObjFusType_FR_Confirm/1 -> Bus Creator/2  "PP_ObjFusType_FR_Confirm"
  Bus Selector1/4 -> AEBLONGTarget_PassedbyTarget/4(AEBLONG_TargetP0_ID_K1)  "<AEBLONG_Target_ID_K1>"
  Object_ID/1 -> Bus Creator/10  "Object_ID"
  PP_ObjFusType_FC_Confirm/1 -> Bus Creator/3  "PP_ObjFusType_FC_Confirm"
  Bus Selector2/1 -> AEBLONGTarget_FusionType/1(PP_ObjFusType_FC_FR_Confirm)  "<PP_ObjFusType_FC_FR_Confirm>"
  Bus Selector1/1 -> AEBLONGTarget_PassedbyTarget/1(FR_Confirm)  "<PP_ObjFusType_FR_Confirm>"
  Bus Selector2/2 -> AEBLONGTarget_FusionType/2(PP_ObjFusType_FR_Confirm)  "<PP_ObjFusType_FC_Confirm>"
  Bus Selector1/5 -> AEBLONGTarget_PassedbyTarget/5(AEBLONG_TargetP0_Dx_K1)  "<AEBLONG_Target_Dx_K1>"
  PP_ObjFusType_FC_FR_Confirm/1 -> Bus Creator/1  "PP_ObjFusType_FC_FR_Confirm"
  Object_DY/1 -> Bus Creator/9  "Object_DY"
  Bus Selector1/2 -> AEBLONGTarget_PassedbyTarget/2(Obj_MovingState)  "<Obj_MovingState>"
  Bus Selector3/2 -> AEBLONGTarget_Fence/2(Obj_MovingState)  "<Obj_MovingState>"
  Obj_MovingState/1 -> Bus Creator/4  "Obj_MovingState"
  Bus Selector1/3 -> AEBLONGTarget_PassedbyTarget/3(Obj_Dx)  "<Obj_Dx>"
  Object_ObstacleProb/1 -> Bus Creator/8  "Object_ObstacleProb"
  Bus Selector3/3 -> AEBLONGTarget_Fence/3(Object_ObstacleProb)  "<Object_ObstacleProb>"
  Bus Selector3/4 -> AEBLONGTarget_Fence/4(Object_DY)  "<Object_DY>"
  Bus Selector3/1 -> AEBLONGTarget_Fence/1(FR_Confirm)  "<PP_ObjFusType_FR_Confirm>"
  Obj_Dx/1 -> Bus Creator/5  "Obj_Dx"
  AEBLONG_Target_ID_K1/1 -> Bus Creator/6  "AEBLONG_Target_ID_K1"
  AEBLONG_Target_Dx_K1/1 -> Bus Creator/7  "AEBLONG_Target_Dx_K1"
  Bus Selector7/1 -> REElementType/1(PP_REElementType)  "<PP_REElementType>"
  REElementType/1(TOS_AEBLONG_Target_REElementType) -> TOS_AEBLONG_Target_REElementType_ObserVale/1, Logical Operator3/4
  Bus Creator/1 -> Bus Selector7/1, Bus Selector3/1, Bus Selector1/1, Bus Selector2/1
  PP_REElementType/1 -> Bus Creator/11  "PP_REElementType"

== system PubIfDecisionTOS_MDL/TOS_20201112/TOS_2012080320/TOS/AEB/TOS_AEBLong/AEBLong_Target_PreJudge/AEBLONG_Target_PreFilt/AEBLONG_TargetPreCondJudgeDefault ==
  Action Port : ActionPort  ActionPortLabel=if(u1 ~= 0)
  Constant{1..5} (5 alike) : Constant  Value=0  OutDataTypeStr=boolean
  TOS_AEBLONG_Target_PreFiltFlag : Outport
  TOS_AEBLONG_Target_FusionTypeFlag_ObserVale : Outport  Port=2
  TOS_AEBLONG_Target_PassedbyTarget_Flag_ObserVale : Outport  Port=3
  TOS_AEBLONG_Target_FenceFlag_ObserVale : Outport  Port=4
  TOS_AEBLONG_Target_REElementType_ObserVale : Outport  Port=5
  wires:
  Constant2/1 -> TOS_AEBLONG_Target_PreFiltFlag/1
  Constant1/1 -> TOS_AEBLONG_Target_FusionTypeFlag_ObserVale/1
  Constant3/1 -> TOS_AEBLONG_Target_PassedbyTarget_Flag_ObserVale/1
  Constant4/1 -> TOS_AEBLONG_Target_FenceFlag_ObserVale/1
  Constant5/1 -> TOS_AEBLONG_Target_REElementType_ObserVale/1
